simulink model "a"  (R2020b)
settings: Solver=VariableStepAuto  StartTime=0.0  StopTime=30  RelTol=1e-3
libraries: cstblocks x2, simulink_extras x1
settings Model: Creator=piero  LastModifiedBy=piero

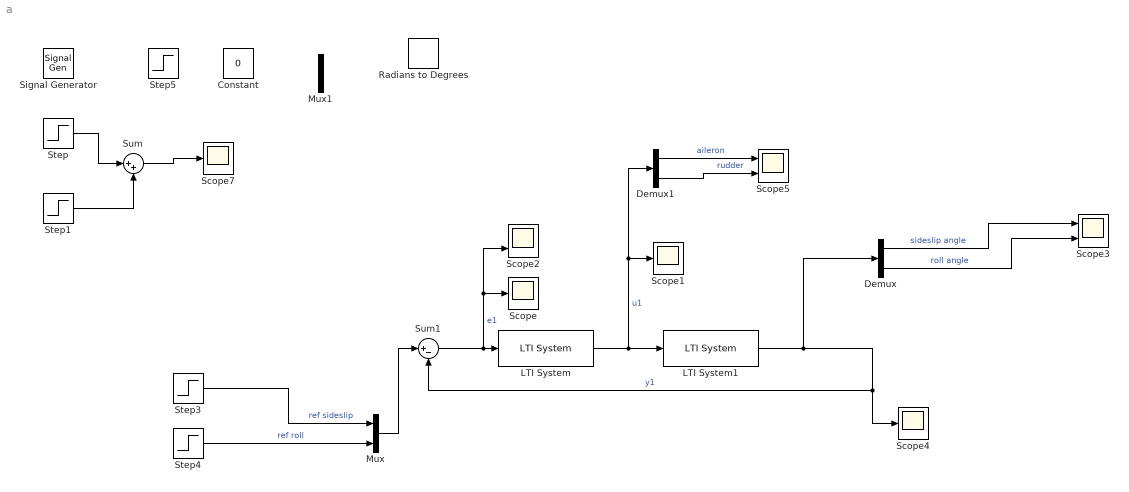
== system a ==
  Constant : Constant  Value=0
  Demux : Demux  Outputs=2
  Demux1 : Demux  Outputs=2
  LTI System : cstblocks/LTI System  sys=K4  IC=[]
  LTI System1 : cstblocks/LTI System  sys=P  IC=[]
  Mux : Mux  Inputs=2
  Mux1 : Mux  Inputs=2
  Radians to Degrees : simulink_extras/Transformations/Radians to Degrees
  Scope{,1,4,7} (4 alike) : Scope
  Scope2 : Scope  NumInputPorts=2
  Scope3 : Scope  NumInputPorts=2
  Scope5 : Scope  NumInputPorts=2
  Signal Generator : SignalGenerator  WaveForm=sawtooth  Amplitude=0.2  Units=rad/sec
  Step : Step  Time=2  After=pi/90  SampleTime=0
  Step1 : Step  Time=6  After=-pi/90  SampleTime=0  ZeroCross=off
  Step3 : Step  Time=2  After=pi/90  SampleTime=0
  Step4 : Step  Time=2  After=pi/6  SampleTime=0
  Step5 : Step  SampleTime=0
  Sum : Sum  Inputs=|++
  Sum1 : Sum  Inputs=|+-
  wires:
  LTI System/1 -> Demux1/1, Scope1/1, LTI System1/1  "u1"
  Sum1/1 -> Scope2/2, Scope/1, LTI System/1  "e1"
  LTI System1/1 -> Scope4/1, Sum1/2, Demux/1  "y1"
  Step/1 -> Sum/1
  Step1/1 -> Sum/2
  Demux/1 -> Scope3/1  "sideslip angle"
  Demux/2 -> Scope3/2  "roll angle"
  Demux1/1 -> Scope5/1  "aileron"
  Demux1/2 -> Scope5/2  "rudder"
  Mux/1 -> Sum1/1
  Sum/1 -> Scope7/1
  Step3/1 -> Mux/1  "ref sideslip"
  Step4/1 -> Mux/2  "ref roll"
